simulink library "inInputDevice"  (R2016b)
settings: Solver=VariableStepAuto  StartTime=0.0  StopTime=10.0  RelTol=1e-3
settings Model: Creator=Nathan  LastModifiedBy=Nathan

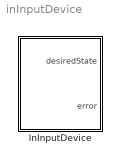
== system inInputDevice ==
  InInputDevice : Subsystem

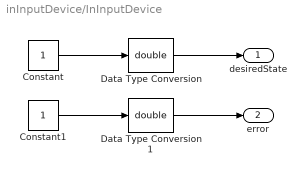
== system inInputDevice/InInputDevice ==
  Constant : Constant
  Constant1 : Constant
  Data Type Conversion : DataTypeConversion  OutDataTypeStr=double
  Data Type Conversion1 : DataTypeConversion  OutDataTypeStr=double
  desiredState : Outport
  error : Outport  Port=2
  wires:
  Constant1/1 -> Data Type Conversion1/1
  Constant/1 -> Data Type Conversion/1
  Data Type Conversion/1 -> desiredState/1
  Data Type Conversion1/1 -> error/1
